simulink model "Digitizing_3delays_1us"  (R2014a)
settings: Solver=FixedStepDiscrete  StartTime=0.0  StopTime=0.0  FixedStep=1  RelTol=1e-3
values from neighbouring files (symbols this model uses):
  inputPulse = inputSequence ( 76*10^6, 1, 0, 0, 300*10^-9)    [generateBus.m]    (also in plotSimulinkOutput_grid.m = inputSequence(76.92307692*10^6, 1, 0,1.5*10^-6); pulseModel.m = [75.76*10^6, 10, 0, 0, 1])
libraries: opticalComponentLibrary x25
settings Model: Creator=Nithya Menon  LastModifiedBy=Nithya Menon

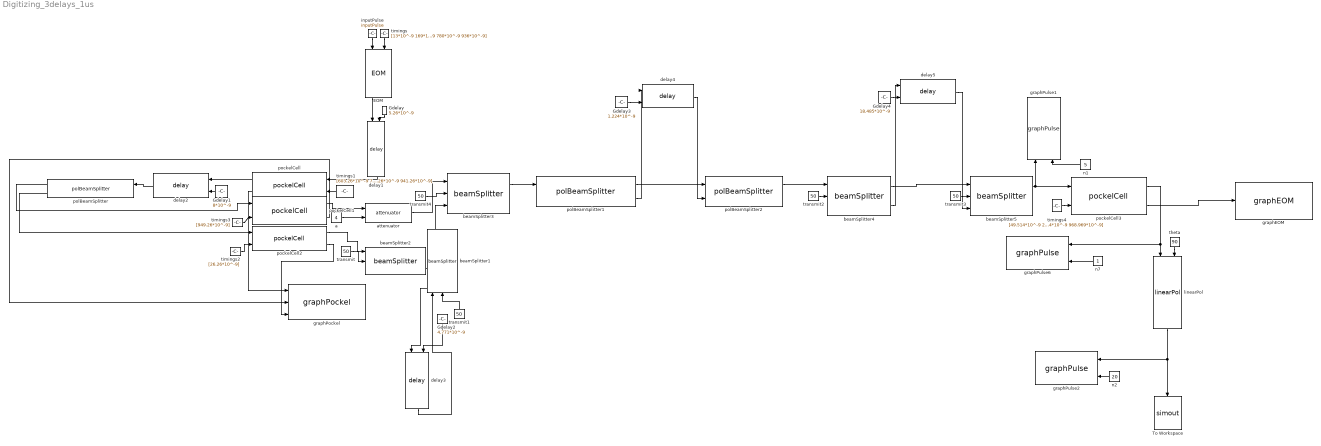
== system Digitizing_3delays_1us ==
  EOM : opticalComponentLibrary/EOM
  Gdelay : Constant  Value=5.26*10^-9
  Gdelay1 : Constant  Value=8*10^-9
  Gdelay2 : Constant  Value=4.771*10^-9
  Gdelay3 : Constant  Value=1.224*10^-9
  Gdelay4 : Constant  Value=18.485*10^-9
  To Workspace : ToWorkspace  VariableName=simout  SampleTime=-1
  a : Constant  Value=4
  attenuator : opticalComponentLibrary/attenuator
  beamSplitter{1..5} (5 alike) : opticalComponentLibrary/beamSplitter
  delay{1..5} (5 alike) : opticalComponentLibrary/delay
  graphEOM : opticalComponentLibrary/graphEOM
  graphPockel : opticalComponentLibrary/graphPockel
  graphPulse1 : opticalComponentLibrary/graphPulse
  graphPulse2 : opticalComponentLibrary/graphPulse
  graphPulse6 : opticalComponentLibrary/graphPulse
  inputPulse : Constant  Value=inputPulse
  linearPol : opticalComponentLibrary/linearPol
  n1 : Constant  Value=5
  n2 : Constant  Value=20
  n7 : Constant
  pockelCell{,1..3} (4 alike) : opticalComponentLibrary/pockelCell
  polBeamSplitter : opticalComponentLibrary/polBeamSplitter
  polBeamSplitter1 : opticalComponentLibrary/polBeamSplitter
  polBeamSplitter2 : opticalComponentLibrary/polBeamSplitter
  theta : Constant  Value=90
  timings : Constant  Value="[13*10^-9 169*10^-9 351*10^-9  598*10^-9 780*10^-9 936*10^-9]"
  timings1 : Constant  Value=[603.26*10^-9 783.26*10^-9 941.26*10^-9]
  timings2 : Constant  Value=[26.26*10^-9]
  timings3 : Constant  Value=[949.26*10^-9]
  timings4 : Constant  Value=[49.514*10^-9 206.739*10^-9 370.254*10^-9 611.26*10^-9 811.744*10^-9 968.969*10^-9]
  transmit{,1..4} (5 alike) : Constant  Value=50
  wires:
  inputPulse/1 -> EOM/1
  timings/1 -> EOM/2
  EOM/1 -> delay1/1
  Gdelay/1 -> delay1/2
  pockelCell/1 -> delay2/1
  Gdelay1/1 -> delay2/2
  delay2/1 -> polBeamSplitter/1
  polBeamSplitter/1 -> pockelCell1/1
  polBeamSplitter/2 -> pockelCell2/1
  pockelCell2/1 -> beamSplitter2/1
  beamSplitter2/2 -> delay3/1
  delay3/1 -> beamSplitter1/1
  Gdelay2/1 -> delay3/2
  transmit/1 -> beamSplitter2/2
  transmit1/1 -> beamSplitter1/2
  timings1/1 -> pockelCell/2
  timings2/1 -> pockelCell2/2
  timings3/1 -> pockelCell1/2
  beamSplitter3/1 -> polBeamSplitter1/1
  polBeamSplitter1/1 -> polBeamSplitter2/1
  polBeamSplitter1/2 -> delay4/1
  Gdelay3/1 -> delay4/2
  delay4/1 -> polBeamSplitter2/2
  transmit2/1 -> beamSplitter4/2
  transmit3/1 -> beamSplitter5/2
  polBeamSplitter2/1 -> beamSplitter4/1
  beamSplitter4/1 -> beamSplitter5/1
  Gdelay4/1 -> delay5/2
  beamSplitter4/2 -> delay5/1
  delay5/1 -> beamSplitter5/3
  beamSplitter5/1 -> graphPulse1/1, pockelCell3/1
  timings4/1 -> pockelCell3/2
  pockelCell3/1 -> linearPol/1, graphPulse6/1
  delay1/1 -> pockelCell/1
  transmit4/1 -> beamSplitter3/2
  beamSplitter1/1 -> beamSplitter3/3
  pockelCell1/1 -> attenuator/1
  attenuator/1 -> beamSplitter3/1
  a/1 -> attenuator/2
  n7/1 -> graphPulse6/2
  pockelCell/2 -> graphPockel/1
  pockelCell1/2 -> graphPockel/2
  pockelCell2/2 -> graphPockel/3
  pockelCell3/2 -> graphEOM/1
  n1/1 -> graphPulse1/2
  linearPol/1 -> graphPulse2/1, To Workspace/1
  theta/1 -> linearPol/2
  n2/1 -> graphPulse2/2
